simulink model "WZ_CAE_4_2"  (R2023b)
settings: Solver=VariableStepAuto  StartTime=0.0  StopTime=10  MaxStep=0.01  RelTol=1e-3
settings Model: Creator=user  LastModifiedBy=Wojciech Zub
settings SolverCC: AlgebraicLoopSolver=TrustRegion
settings DebuggingCC: UnconnectedInputMsg=warning  UnconnectedOutputMsg=warning  UnconnectedLineMsg=warning
settings ModelReferenceCC: EnableRefExpFcnMdlSchedulingChecks=on

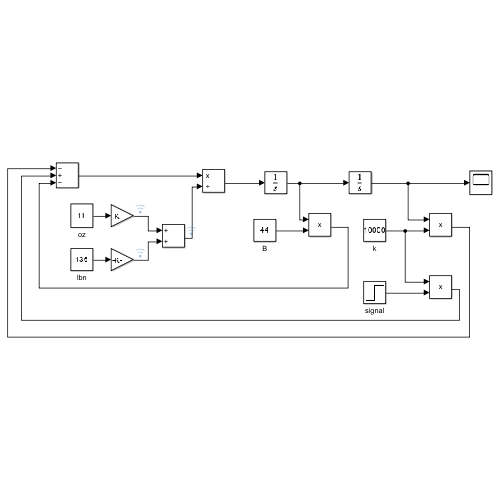
[thumbnail: Simulink's stored preview of the top-level diagram]
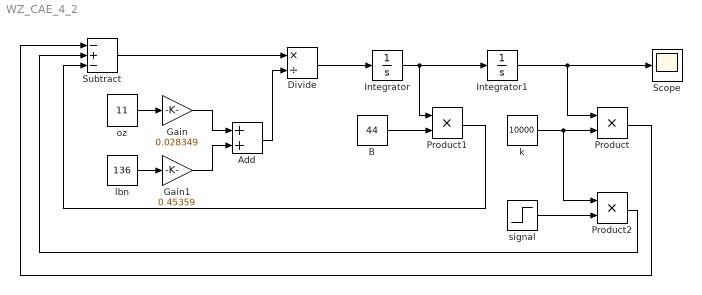
== system WZ_CAE_4_2 ==
  Add : Sum
  B : Constant  Value=44
  Divide : Product  Inputs=*/
  Gain : Gain  Gain=0.028349
  Gain1 : Gain  Gain=0.45359
  Integrator : Integrator
  Integrator1 : Integrator
  Product : Product
  Product1 : Product
  Product2 : Product
  Scope : Scope
  Subtract : Sum  Inputs=-+-
  k : Constant  Value=10000
  lbn : Constant  Value=136
  oz : Constant  Value=11
  signal : Step  Time=0.01  SampleTime=0
  wires:
  signal/1 -> Product2/2
  Gain1/1 -> Add/2
  lbn/1 -> Gain1/1
  Gain/1 -> Add/1
  oz/1 -> Gain/1
  Add/1 -> Divide/2
  k/1 -> Product2/1, Product/2
  B/1 -> Product1/2
  Integrator/1 -> Integrator1/1, Product1/1
  Divide/1 -> Integrator/1
  Product/1 -> Subtract/1
  Subtract/1 -> Divide/1
  Integrator1/1 -> Scope/1, Product/1
  Product2/1 -> Subtract/2
  Product1/1 -> Subtract/3
